simulink model "S_shape_TuningMethod"  (R2023b)
settings: Solver=VariableStepAuto  StartTime=0.0  StopTime=10.0  RelTol=1e-3
values from neighbouring files (symbols this model uses):
  den = conv([1 2], [1 5])    [S_shape.m]
  Kd = Kp * Td    [S_shape.m]
  Ki = Kp / Ti    [S_shape.m]
  Kp = (1.2*T)/K*L    [S_shape.m]
  num = [1]    [S_shape.m]
settings Model: Creator=MOHAMED  LastModifiedBy=MOHAMED

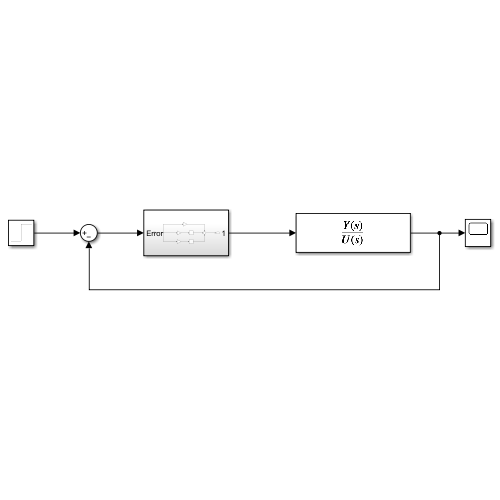
[thumbnail: Simulink's stored preview of the top-level diagram]
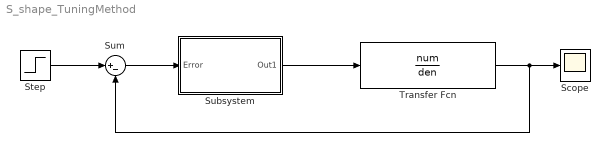
== system S_shape_TuningMethod ==
  Scope : Scope
  Step : Step  SampleTime=0
  Subsystem : Subsystem
  Sum : Sum  Inputs=|+-
  Transfer Fcn : TransferFcn  Numerator=num  Denominator=den
  wires:
  Transfer Fcn/1 -> Sum/2, Scope/1
  Step/1 -> Sum/1
  Sum/1 -> Subsystem/1(Error)
  Subsystem/1(Out1) -> Transfer Fcn/1

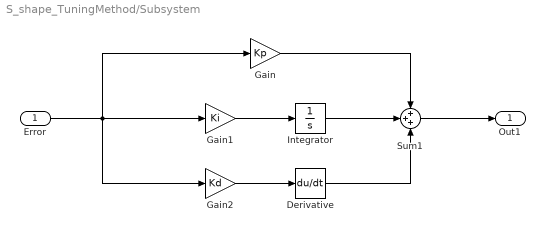
== system S_shape_TuningMethod/Subsystem ==
  Error : Inport
  Derivative : Derivative
  Gain : Gain  Gain=Kp
  Gain1 : Gain  Gain=Ki
  Gain2 : Gain  Gain=Kd
  Integrator : Integrator
  Sum1 : Sum  Inputs=+++
  Out1 : Outport
  wires:
  Gain2/1 -> Derivative/1
  Integrator/1 -> Sum1/2
  Gain1/1 -> Integrator/1
  Error/1 -> Gain2/1, Gain1/1, Gain/1
  Derivative/1 -> Sum1/3
  Sum1/1 -> Out1/1
  Gain/1 -> Sum1/1
